simulink model "AlmostFinishedObserverBlock2016a"  (R2016a)
settings: Solver=VariableStepAuto  SolverMode=SingleTasking  StartTime=0.0  StopTime=10.0  RelTol=1e-3
undefined symbols (not defined in the file): M, RTransposed
libraries: marine_gnc x2
settings Model: Creator=simen  LastModifiedBy=simen
settings DataIOCC: ReturnWorkspaceOutputs=on
settings DebuggingCC: SFUnexpectedBacktrackingDiag=error  SFNoUnconditionalDefaultTransitionDiag=error
settings SFSimCC: SimUseLocalCustomCode=on
settings RTWCC: RTWUseLocalCustomCode=on
settings GRTTargetCC: TargetLangStandard=C99 (ISO)  GeneratePreprocessorConditionals=Use local settings
settings ConfigComp: CovMetricSettings=dwe  CovHtmlReporting=off  CovSaveCumulativeToWorkspaceVar=off  CovSaveSingleToWorkspaceVar=off  CovExternalEMLEnable=on

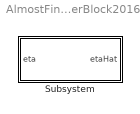
== system AlmostFinishedObserverBlock2016a ==
  Subsystem : Subsystem

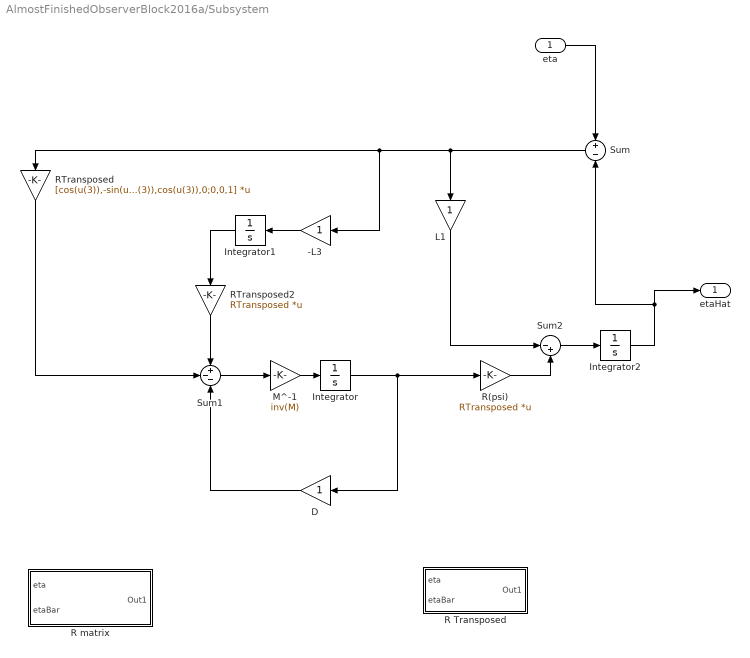
== system AlmostFinishedObserverBlock2016a/Subsystem ==
  eta : Inport
  -L3 : Gain
  D : Gain
  Integrator : Integrator
  Integrator1 : Integrator
  Integrator2 : Integrator
  L1 : Gain
  M^-1 : Gain  Gain=inv(M)
  R Transposed : Subsystem
  "R matrix " : Subsystem
  R(psi) : Gain  Gain=RTransposed  Multiplication=Matrix(K*u)
  RTransposed : Gain  Gain=[cos(u(3)),-sin(u(3)),0;sin(u(3)),cos(u(3)),0;0,0,1]  Multiplication=Matrix(K*u)
  RTransposed2 : Gain  Gain=RTransposed  Multiplication=Matrix(K*u)
  Sum : Sum  Inputs=+|-
  Sum1 : Sum  Inputs=+--
  Sum2 : Sum  Inputs=|-+
  etaHat : Outport
  wires:
  Sum/1 -> L1/1, -L3/1, RTransposed/1
  eta/1 -> Sum/1
  M^-1/1 -> Integrator/1
  RTransposed/1 -> Sum1/2
  Sum1/1 -> M^-1/1
  D/1 -> Sum1/3
  RTransposed2/1 -> Sum1/1
  Integrator1/1 -> RTransposed2/1
  -L3/1 -> Integrator1/1
  Integrator/1 -> R(psi)/1, D/1
  R(psi)/1 -> Sum2/2
  L1/1 -> Sum2/1
  Sum2/1 -> Integrator2/1
  Integrator2/1 -> etaHat/1, Sum/2

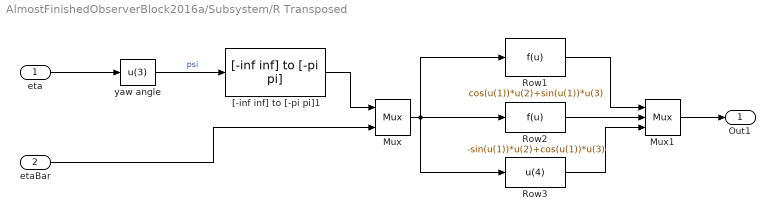
== system AlmostFinishedObserverBlock2016a/Subsystem/R Transposed ==
  eta : Inport
  etaBar : Inport  Port=2
  Mux : Mux  Inputs=2
  Mux1 : Mux  Inputs=3
  Row1 : Fcn  Expr=cos(u(1))*u(2)+sin(u(1))*u(3)
  Row2 : Fcn  Expr=-sin(u(1))*u(2)+cos(u(1))*u(3)
  Row3 : Fcn  Expr=u(4)
  "[-inf inf] to [-pi pi]1" : marine_gnc/Utilities/Math Operations/[-inf inf] to [-pi pi]
  yaw angle : Fcn  Expr=u(3)
  Out1 : Outport
  wires:
  Mux1/1 -> Out1/1
  etaBar/1 -> Mux/2
  Mux/1 -> Row3/1, Row2/1, Row1/1
  Row1/1 -> Mux1/1
  Row3/1 -> Mux1/3
  Row2/1 -> Mux1/2
  "[-inf inf] to [-pi pi]1"/1 -> Mux/1
  eta/1 -> yaw angle/1
  yaw angle/1 -> "[-inf inf] to [-pi pi]1"/1  "psi"

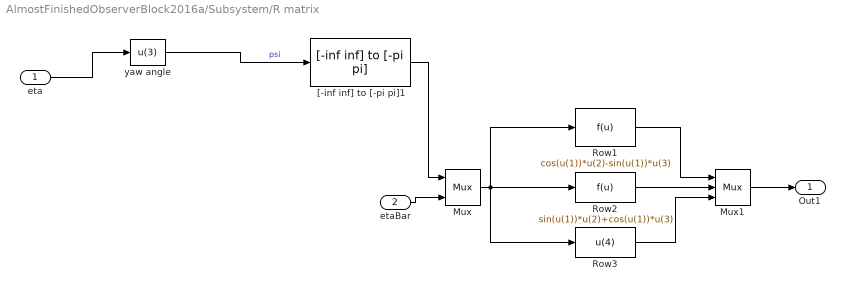
== system AlmostFinishedObserverBlock2016a/Subsystem/R matrix  ==
  eta : Inport
  etaBar : Inport  Port=2
  Mux : Mux  Inputs=2
  Mux1 : Mux  Inputs=3
  Row1 : Fcn  Expr=cos(u(1))*u(2)-sin(u(1))*u(3)
  Row2 : Fcn  Expr=sin(u(1))*u(2)+cos(u(1))*u(3)
  Row3 : Fcn  Expr=u(4)
  "[-inf inf] to [-pi pi]1" : marine_gnc/Utilities/Math Operations/[-inf inf] to [-pi pi]
  yaw angle : Fcn  Expr=u(3)
  Out1 : Outport
  wires:
  Mux1/1 -> Out1/1
  etaBar/1 -> Mux/2
  Mux/1 -> Row3/1, Row2/1, Row1/1
  Row1/1 -> Mux1/1
  Row3/1 -> Mux1/3
  Row2/1 -> Mux1/2
  "[-inf inf] to [-pi pi]1"/1 -> Mux/1
  eta/1 -> yaw angle/1
  yaw angle/1 -> "[-inf inf] to [-pi pi]1"/1  "psi"
